simulink library "solarPressure_lib"  (R2018b)
settings: Solver=VariableStepAuto  StartTime=0.0  StopTime=10.0  RelTol=1e-3
undefined symbols (not defined in the file or in its folder): simParams
libraries: vrlib x1, aerolibutil x1, sunVectorEclipse_lib x1
settings Model: Creator=devantormey  LastModifiedBy=Taylor

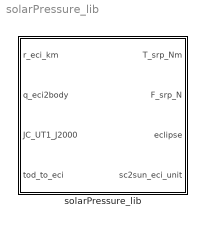
== system solarPressure_lib ==
  solarPressure_lib : Subsystem

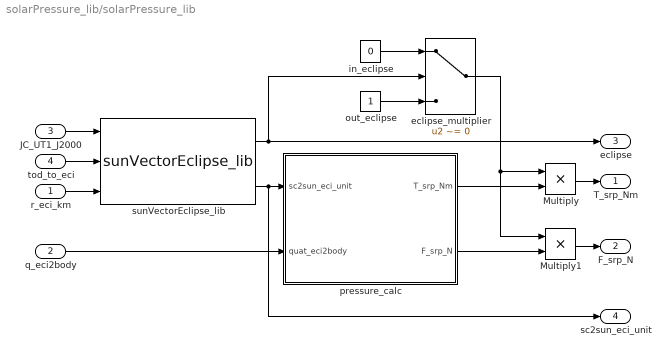
== system solarPressure_lib/solarPressure_lib ==
  r_eci_km : Inport
  q_eci2body : Inport  Port=2
  JC_UT1_J2000 : Inport  Port=3
  tod_to_eci : Inport  Port=4
  Multiply : Product
  Multiply1 : Product
  eclipse_multiplier : Switch  Criteria=u2 ~= 0
  in_eclipse : Constant  Value=0  OutDataTypeStr=boolean
  out_eclipse : Constant  OutDataTypeStr=boolean
  pressure_calc : Subsystem
  sunVectorEclipse_lib : sunVectorEclipse_lib/sunVectorEclipse_lib  SystemSampleTime=-1
  T_srp_Nm : Outport
  F_srp_N : Outport  Port=2
  eclipse : Outport  Port=3
  sc2sun_eci_unit : Outport  Port=4
  wires:
  sunVectorEclipse_lib/2 -> sc2sun_eci_unit/1, pressure_calc/1(sc2sun_eci_unit)
  pressure_calc/2(F_srp_N) -> Multiply1/2
  pressure_calc/1(T_srp_Nm) -> Multiply/2
  q_eci2body/1 -> pressure_calc/2(quat_eci2body)
  JC_UT1_J2000/1 -> sunVectorEclipse_lib/1
  tod_to_eci/1 -> sunVectorEclipse_lib/2
  r_eci_km/1 -> sunVectorEclipse_lib/3
  Multiply1/1 -> F_srp_N/1
  Multiply/1 -> T_srp_Nm/1
  sunVectorEclipse_lib/1 -> eclipse_multiplier/2, eclipse/1
  in_eclipse/1 -> eclipse_multiplier/1
  eclipse_multiplier/1 -> Multiply1/1, Multiply/1
  out_eclipse/1 -> eclipse_multiplier/3

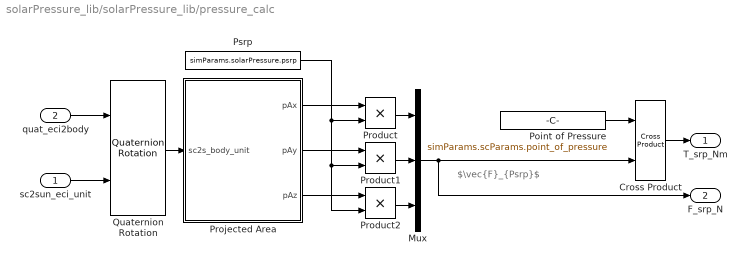
== system solarPressure_lib/solarPressure_lib/pressure_calc ==
  note: $\vec{F}_{Psrp}$
  sc2sun_eci_unit : Inport
  quat_eci2body : Inport  Port=2
  Cross Product : vrlib/Utilities/Cross Product
      settings: SourceProductBaseCode=VR
  Mux : Mux  Inputs=3
  Point of Pressure : Constant  Value=simParams.scParams.point_of_pressure
  Product : Product
  Product1 : Product
  Product2 : Product
  Projected Area : Subsystem
  Psrp : Constant  Value=simParams.solarPressure.psrp
  Quaternion Rotation : aerolibutil/Quaternion Rotation
  T_srp_Nm : Outport
  F_srp_N : Outport  Port=2
  wires:
  Psrp/1 -> Product/2, Product1/2, Product2/2
  Projected Area/2(pAy) -> Product1/1
  Projected Area/3(pAz) -> Product2/1
  Product/1 -> Mux/1
  Product1/1 -> Mux/2
  Product2/1 -> Mux/3
  Point of Pressure/1 -> Cross Product/1
  Cross Product/1 -> T_srp_Nm/1
  Quaternion Rotation/1 -> Projected Area/1(sc2s_body_unit)
  Projected Area/1(pAx) -> Product/1
  quat_eci2body/1 -> Quaternion Rotation/1
  Mux/1 -> F_srp_N/1, Cross Product/2
  sc2sun_eci_unit/1 -> Quaternion Rotation/2

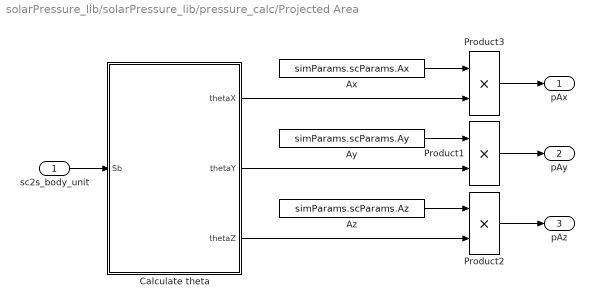
== system solarPressure_lib/solarPressure_lib/pressure_calc/Projected Area ==
  sc2s_body_unit : Inport
  Ax : Constant  Value=simParams.scParams.Ax
  Ay : Constant  Value=simParams.scParams.Ay
  Az : Constant  Value=simParams.scParams.Az
  Calculate theta : MATLAB Function  TreatAsAtomicUnit=on
  Product1 : Product
  Product2 : Product
  Product3 : Product
  pAx : Outport
  pAy : Outport  Port=2
  pAz : Outport  Port=3
  wires:
  Product1/1 -> pAy/1
  Product2/1 -> pAz/1
  Az/1 -> Product2/1
  Calculate theta/3(thetaZ) -> Product2/2
  Ay/1 -> Product1/1
  Calculate theta/1(thetaX) -> Product3/2
  Calculate theta/2(thetaY) -> Product1/2
  Product3/1 -> pAx/1
  sc2s_body_unit/1 -> Calculate theta/1(Sb)
  Ax/1 -> Product3/1

== matlab function solarPressure_lib/pressure_calc/Projected Area/Calculate theta ==
  data: Sb input; thetaX output; thetaY output; thetaZ output
% Author: Devan Tormey
% Date: 2/21/2019
function [thetaX,thetaY,thetaZ] = fcn(Sb)
%#codegen
% Description: This function computes the dot product of the sun vector
% with the appropriate body coordinate vector.
%~~~~~~~~~~~~~ 
%  Variables 
%~~~~~~~~~~~~~~
% Sb - this is the sun vector (calculated elsewhere)
% ThetaXYZ - as these are all unit vectors the dot product produces the
% cosine of the angle in between

    if Sb(1) >= 0 
        thetaX = dot(Sb,[1;0;0]);
    else 
        thetaX = dot(Sb,[-1;0;0]);
    end

    if Sb(2) >= 0 
        thetaY = dot(Sb,[0;1;0]);
    else 
        thetaY = dot(Sb,[0;-1;0]);
    end

    if Sb(3) >= 0 
        thetaZ = dot(Sb,[0;0;1]);
    else 
        thetaZ = dot(Sb,[0;0;-1]);
    end

end
